simulink model "OWC_rigid"  (R2021b)
settings: Solver=ode45  StartTime=0  StopTime=500  FixedStep=0.01  MaxStep=0.01  RelTol=1e-3  EnableMultiTasking=on
values from neighbouring files (symbols this model uses):
  controlTimestep = 5    [wecSimInputFile.m]
  fExcTimestep = .05    (= 0.05)    [wecSimInputFile.m]
  simu = simulationClass()    [wecSimInputFile.m]
  Z = waveAmplitude * sin(waveFrequency * X) .* cos(waveFrequency * Y)    [userDefinedFunctions.m]
undefined symbols (not defined in the file or in its folder): airChamber, body, constraint, geometry, hydroData, MoorDyn, mooring, pto, turb, WECSim_Lib_Moorings, X, Y
libraries: simulink x6, sm_lib x5, WECSim_Lib_Body_Elements x3, nesl_utility x2, WECSim_Lib_Constraints x1, WECSim_Lib_Frames x1, WECSim_Lib_PTOs x1
settings Model: Creator=mlawson  LastModifiedBy=mshabara
settings SolverCC: ZeroCrossControl=DisableAll  AlgebraicLoopSolver=LineSearch  AutoInsertRateTranBlk=on
settings DataIOCC: SaveFormat=Array  SaveOutput=off  SaveTime=off  ReturnWorkspaceOutputs=off
settings OptimizationCC: LifeSpan=inf  SimCompilerOptimization=on
settings DebuggingCC: MergeDetectMultiDrivingBlocksExec=none  SolverPrmCheckMsg=warning  AllowSymbolicDim=off  StateNameClashWarn=warning  SFUnexpectedBacktrackingDiag=warning  SFNoUnconditionalDefaultTransitionDiag=warning  SFExecutionAtInitializationDiag=none  ArithmeticOperatorsInVariantConditions=warning
settings HardwareCC: ProdBitPerPointer=32  ProdBitPerSizeT=32  ProdBitPerPtrDiffT=32  ProdLargestAtomicFloat=None  ProdIntDivRoundTo=Undefined  ProdEndianess=Unspecified  ProdWordSize=32  ProdHWDeviceType=32-bit Generic
settings ModelReferenceCC: PropagateSignalLabelsOutOfModel=off
settings SFSimCC: SimUseLocalCustomCode=off  CustomCodeUndefinedFunction=UseInterfaceOnly
settings RTWCC: RTWUseLocalCustomCode=off  DLArmComputeVersion=20.02.1
settings CodeAppCC: StateflowObjectComments=on
settings GRTTargetCC: TargetLangStandard=C89/C90 (ANSI)
settings ConfigComp: CovMetricSettings=dw  CovSaveCumulativeToWorkspaceVar=on  CovSaveSingleToWorkspaceVar=on  CovExternalEMLEnable=off  CovSFcnEnable=off
settings SimscapeCC: SimscapeNormalizeSystem=off
settings ConfigurationSet: Description=SimMechanics 2G
settings ExplorerConfigSet: SimMechanicsOpenEditorOnUpdate=off  InternalSimMechanicsExplorerSettings="<ExplorerConfiguration><canonicalview>default</canonicalview><TilePanel><TileInfo><Tiles Columns=\"1\" Count=\"1\" Rows=\"1\"><Column Left=\"2\" Weight=\"1\"/><Column Left=\"1335\"/><Row Top=\"2\" Weight=\"1\"/><Row Top=\"911\"/><Tile Height=\"1\" Width=\"1\" X=\"0\" Y=\"0\"/></Tiles></TileInfo><SceneInfo><SceneViewer><BGColor><R>0.60000002384185791</R><G>0.60000002384185791</G><B>0.60000002384185791</B></BGColor><Camera><Position><X>365.37645888990272</X><Y>-369.82486814446582</Y><Z>359.64809521743916</Z></Position><Center><X>-6.7351450971904585</X><Y>2.2867358426280204</Y><Z>-12.463508769654169</Z></Center><Up><X>-0.40824829046386307</X><Y>0.40824829046386307</Y><Z>0.81649658092772615</Z></Up><Left>-57.820127362122818</Left><Right>57.820127362122818</Right><Bottom>-38.308817187253304</Bottom><Top>38.308817187253304</Top></Camera></SceneViewer></SceneInfo></TilePanel></ExplorerConfiguration>"

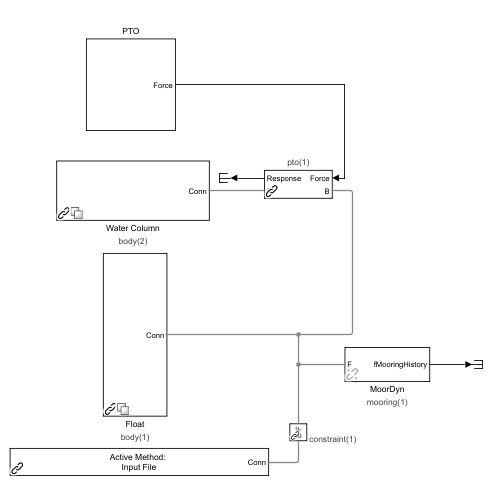
[thumbnail: Simulink's stored preview of the top-level diagram]
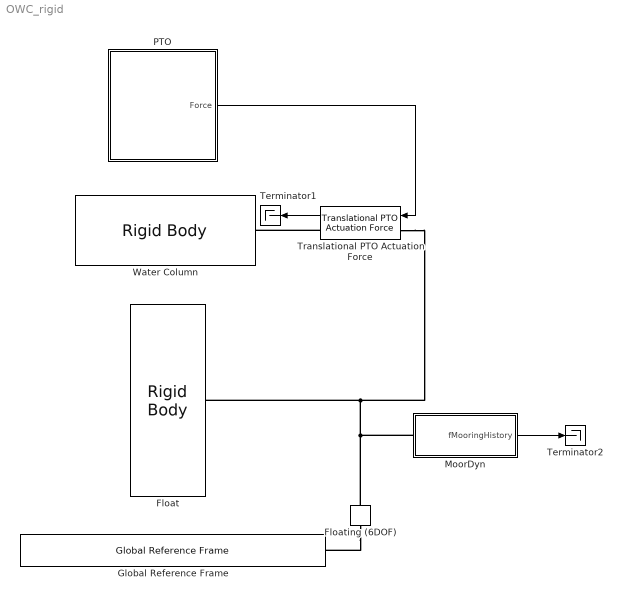
== system OWC_rigid ==
  Float : WECSim_Lib_Body_Elements/Rigid Body  body=body(1)  h5File=hydroData/*.h5  geometryFile=geometry/*.stl  mass=0  inertia=0 0 0  inertiaProducts=0 0 0  nonHydro=0  nonlinearHydro=0  centerGravity=0 0 0  centerBuoyancy=0 0 0  dof=6  volume=0  QTFs=0  displacement=0 0 0  axis=0 1 0  angle=0  option=0  cd=0 0 0  ca=0 0 0  area=0 0 0  VME=0  rgME=0 0 0  z=0 0 1
      settings: SourceProductName=WEC-Sim
  Floating (6DOF) : WECSim_Lib_Constraints/Floating (6DOF)  constraint=constraint(1)  loc="0  0  0"  displacement=0 0 0  y=0 1 0  z=0 0 1  upperLimitSpecify=off  upperLimitBound=0  upperLimitTransitionRegionWidth=0  upperLimitStiffness=0  upperLimitDamping=0  lowerLimitSpecify=off  lowerLimitBound=0  lowerLimitTransitionRegionWidth=0  lowerLimitStiffness=0  lowerLimitDamping=0
      settings: AttributesFormatString=%<constraint>
  Global Reference Frame : WECSim_Lib_Frames/Global Reference Frame  waves=waves  simu=simu  InputMethod=Input File  InputFile=wecSimInputFile.m  mode=normal  explorer=off  solver=ode4  startTime=0  rampTime=100  endTime=400  dt=0.1  cicEndTime=60  stateSpace=0  WaveClass=regular  height=2.5  period=8  elevationFile=NOT DEFINED  spectrumFile=NOT DEFINED  direction=0  spread=1  spectrumType=NOT DEFINED  phaseSeed=0  option=EqualEnergy
      settings: SourceProductName=WEC-Sim
  MoorDyn : Subsystem  AncestorBlock=WECSim_Lib_Moorings/MoorDyn  mask(MoorDyn){mooring=mooring(1), InputFileText=Global Reference Frame option "Use Input File" is selected., MooringRef=0  0  0, moorDynNodes=0, moorDynLines=0}
      mask prompts: mooring "Mooring Name:"; MooringRef "Reference Location [m]:"; moorDynNodes "Number of MoorDyn Nodes:"; moorDynLines "Number of MoorDyn Lines:"
      mask help:
      | A mooring body that applies stiffness, damping and pretensions forces to the follower using a MoorDyn simulation. The response of the mooring body is relative to the global reference frame.
      |
      | The variable name input below must be 'mooring(i)' where i=1,2,...
      | mooring(i) must be defined in the input file with the following fields:
      |
      |     .name (required)
      |             String.
      |             Mooring name. Must comply with Matlab's variable naming rules.
      |     .location (optional)
      |             3x1 vector [x y z] in meters.
      |             Mooring location. Default = [0 0 0]
      |     .initial (optional)
      |             Struct
      |             Contains the initial position, angle and axis of the mooring body.
      |     .initial.displacement (optional)
      |             3x1 vector [x y z] in meters.
      |             Initial linear displacement from the ref position. Default = [0 0 0]
      |             This can can be set directly or with the setInitDisp() method.
      |     .initial.axis (optional)
      |             3x1 vector [x y z]
      |             Initial angular displacement axis. Default = [0 1 0]
      |             This can can be set directly or with the setInitDisp() method.
      |     .initial.angle (optional)
      |             Float.
      |             Initial angular displacement angle about axis in radians. Default = [0 0 0]
      |             This can can be set directly or with the setInitDisp() method.
      |     .moorDynLines (optional)
      |             Float.
      |             Number of lines for MoorDyn to use. Default = 0
      |     .moorDynNodes (optional)
      |             moorDynLines x 1 vector.
      |             Specifies the number of nodes per line in MoorDyn. Default = []
      mask init:
      | if exist('mooring','var')
      |     % toWorkSpace: outputs
      |     h=[gcb '/To Workspace'];
      |     responseName=['mooring' num2str(mooring.number) '_out'];
      |     set_param(h,'VariableName',responseName);
      | end
      | mooring.moorDyn = 1;
      settings: AttributesFormatString=%<mooring>
      mask Help:
      | A mooring body that applies stiffness, damping and pretensions forces to the follower using a MoorDyn simulation. The response of the mooring body is relative to the global reference frame.
      | 
      | The variable name input below must be 'mooring(i)' where i=1,2,...
      | mooring(i) must be defined in the input file with the following fields:
      | 
      |     .name (required)
      |             String.
      |             Mooring name. Must comply with Matlab's variable naming rules.
      |     .location (optional)
      |             3x1 vector [x y z] in meters.
      |             Mooring location. Default = [0 0 0]
      |     .initial (optional)
      |             Struct
      |             Contains the initial position, angle and axis of the mooring body.
      |     .initial.displacement (optional)
      |             3x1 vector [x y z] in meters.
      |             Initial linear displacement from the ref position. Default = [0 0 0]
      |             This can can be set directly or with the setInitDisp() method.
      |     .initial.axis (optional)
      |             3x1 vector [x y z]
      |             Initial angular displacement axis. Default = [0 1 0]
      |             This can can be set directly or with the setInitDisp() method.
      |     .initial.angle (optional)
      |             Float.
      |             Initial angular displacement angle about axis in radians. Default = [0 0 0]
      |             This can can be set directly or with the setInitDisp() method.
      |     .moorDynLines (optional)
      |             Float.
      |             Number of lines for MoorDyn to use. Default = 0
      |     .moorDynNodes (optional)
      |             moorDynLines x 1 vector.
      |             Specifies the number of nodes per line in MoorDyn. Default = []
      mask DialogControl InputFileGroup Prompt: Input File
      mask DialogControl CustomParameterGroup Prompt: Custom Parameters
  PTO : Subsystem
  Terminator1 : Terminator
  Terminator2 : Terminator
  Translational PTO Actuation Force : WECSim_Lib_PTOs/Translational PTO Actuation Force  pto=pto(1)  loc="0  0  0"  stiffness=0  damping=0  equilibriumPosition=0  pretension=0  displacement=0 0 0  y=0 1 0  z=0 0 1  upperLimitSpecify=off  upperLimitBound=0  upperLimitTransitionRegionWidth=0  upperLimitStiffness=0  upperLimitDamping=0  lowerLimitSpecify=off  lowerLimitBound=0  lowerLimitTransitionRegionWidth=0  lowerLimitStiffness=0  lowerLimitDamping=0
      settings: AttributesFormatString=%<pto>
  Water Column : WECSim_Lib_Body_Elements/Rigid Body  body=body(2)  h5File=hydroData/*.h5  geometryFile=geometry/*.stl  mass=0  inertia=0 0 0  inertiaProducts=0 0 0  nonHydro=0  nonlinearHydro=0  centerGravity=0 0 0  centerBuoyancy=0 0 0  dof=6  volume=0  QTFs=0  displacement=0 0 0  axis=0 1 0  angle=0  option=0  cd=0 0 0  ca=0 0 0  area=0 0 0  VME=0  rgME=0 0 0  z=0 0 1
      settings: SourceProductName=WEC-Sim
  wires:
  MoorDyn/1(fMooringHistory) -> Terminator2/1
  Translational PTO Actuation Force/1 -> Terminator1/1
  PTO/1(Force) -> Translational PTO Actuation Force/1
  connections:
  Floating (6DOF)/LConn1 -- Global Reference Frame/RConn1
  MoorDyn/LConn1 -- Floating (6DOF)/RConn1 -- Translational PTO Actuation Force/LConn1 -- Float/RConn1
  Translational PTO Actuation Force/RConn1 -- Water Column/RConn1

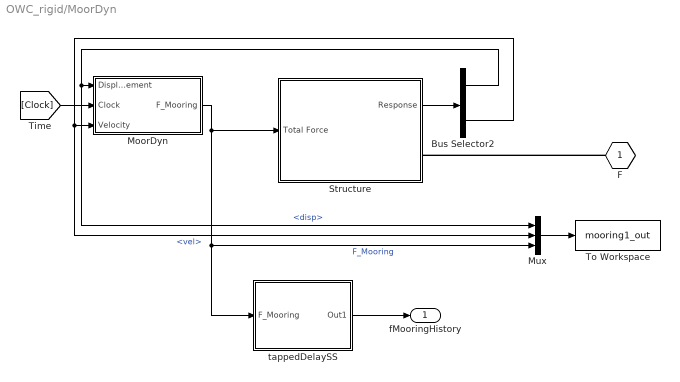
== system OWC_rigid/MoorDyn ==
  Bus Selector2 : BusSelector  OutputSignals=disp,vel
  MoorDyn : Subsystem  VariantControl=sv_moorDyn
  Mux : Mux  Inputs=3
  Structure : Subsystem
  To Workspace : ToWorkspace  VariableName=mooring1_out  SaveFormat=Structure With Time  SampleTime=simu.dtOut
  tappedDelaySS : Subsystem
  F : PMIOPort  Side=Left
  fMooringHistory : Outport
  wires:
  Mux/1 -> To Workspace/1
  Bus Selector2/2 -> MoorDyn/3(Velocity), Mux/2  "<vel>"
  Bus Selector2/1 -> MoorDyn/1(Displacement), Mux/1  "<disp>"
  [Clock] -> MoorDyn/2(Clock)
  MoorDyn/1(F_Mooring) -> Structure/1(Total Force), tappedDelaySS/1(F_Mooring), Mux/3  "F_Mooring"
  Structure/1(Response) -> Bus Selector2/1
  tappedDelaySS/1(Out1) -> fMooringHistory/1
  connections:
  F/RConn1 -- Structure/RConn1

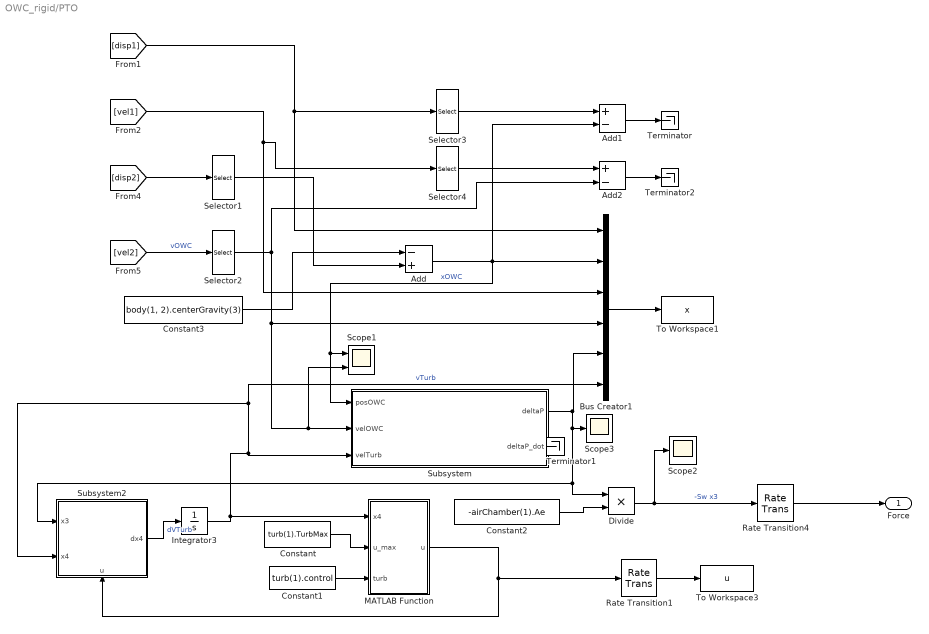
== system OWC_rigid/PTO ==
  Add : Sum  Inputs=-+
  Add1 : Sum  Inputs=+-
  Add2 : Sum  Inputs=+-
  Bus Creator1 : BusCreator  Inputs=6
  Constant : Constant  Value=turb(1).TurbMax
  Constant1 : Constant  Value=turb(1).control
  Constant2 : Constant  Value=-airChamber(1).Ae
  Constant3 : Constant  Value=body(1, 2).centerGravity(3)
  Divide : Product  Inputs=**
  Integrator3 : Integrator  InitialCondition=150
  MATLAB Function : MATLAB Function  TreatAsAtomicUnit=on
  Rate Transition1 : RateTransition  OutPortSampleTimeOpt=Inherit  OutPortSampleTime=controlTimestep
  Rate Transition4 : RateTransition  OutPortSampleTimeOpt=Inherit  OutPortSampleTime=controlTimestep
  Scope1 : Scope  NumInputPorts=2
  Scope2 : Scope
  Scope3 : Scope
  Selector{1..4} (4 alike) : Selector  InputPortWidth=6  IndexOptions=Index vector (dialog)  Indices=3  OutputSizes=1
  Subsystem : Subsystem
  Subsystem2 : Subsystem
      settings: PortSchema="{\"entries\":[{\"content\":{\"sides\":[{\"content\":{\"connectorIds\":[\"In1\",\"In2\"]},\"type\":\"ConnectorPlacement.EquallySpacedRectSide\",\"uuid\":\"efec6f39-391f-477f-a643-1e99d464e6c9\"},{\"content\":{\"connectorIds\":[\"Out1\"],\"side\":\"RIGHT\"},\"type\":\"ConnectorPlacement.EquallySpacedRectSide\",\"uuid\":\"68a722c2-da75-45d7-a9d9-103b5c3e9ffd\"},{\"content\":{\"side\":\"TOP\"},\"type\":\"ConnectorPlacement.EquallySpacedRectSide\",\"uuid\":\"48f59770-5dc2-4659-ad88-cf2781bc51ce\"},{\"content\":{\"connectorIds\":[\"In3\"],\"side\":\"BOTTOM\"},\"type\":\"ConnectorPlacement.EquallySpacedRectSide\",\"uuid\":\"c0a46e7f-e317-4642-bc2a-fe57f83b9e65\"}]},\"type\":\"ConnectorPlacement.EquallySpacedConnector\",\"uuid\":\"2c5b99db-9399-4220-bed2-b879f6d394f4\"}],\"packageUris\":[\"http://schema.mathworks.com/mf0/Connector/R2020b\"],\"version\":\"1.0\"}"
  Terminator : Terminator
  Terminator1 : Terminator
  Terminator2 : Terminator
  To Workspace1 : ToWorkspace  VariableName=x  SaveFormat=Timeseries  SampleTime=-1
  To Workspace3 : ToWorkspace  VariableName=u  SaveFormat=Timeseries  SampleTime=-1
  Force : Outport
  wires:
  Divide/1 -> Scope2/1, Rate Transition4/1  "-Sw x3"
  Add1/1 -> Terminator/1
  [vel1] -> Bus Creator1/3, Selector4/1
  Bus Creator1/1 -> To Workspace1/1
  Constant3/1 -> Add/1
  Add2/1 -> Terminator2/1
  Constant1/1 -> MATLAB Function/3(turb)
  Constant/1 -> MATLAB Function/2(u_max)
  [disp1] -> Bus Creator1/1, Selector3/1
  Subsystem2/1(dx4) -> Integrator3/1  "dVTurb"
  [vel2] -> Selector2/1  "vOWC"
  [disp2] -> Selector1/1
  Integrator3/1 -> Bus Creator1/6, Subsystem2/2(x4), Subsystem/3(velTurb), MATLAB Function/1(x4)  "vTurb"
  Selector3/1 -> Add1/1
  Rate Transition4/1 -> Force/1
  Selector4/1 -> Add2/1
  Add/1 -> Subsystem/1(posOWC), Scope1/1, Add1/2, Bus Creator1/2  "xOWC"
  Subsystem/1(deltaP) -> Scope3/1, Divide/1, Subsystem2/1(x3), Bus Creator1/5
  Subsystem/2(deltaP_dot) -> Terminator1/1
  Constant2/1 -> Divide/2
  Selector1/1 -> Add/2
  Selector2/1 -> Add2/2, Bus Creator1/4, Scope1/2, Subsystem/2(velOWC)
  Rate Transition1/1 -> To Workspace3/1
  MATLAB Function/1(u) -> Rate Transition1/1, Subsystem2/3(u)

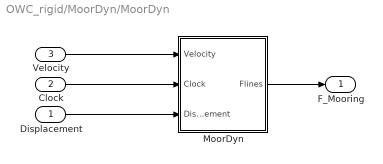
== system OWC_rigid/MoorDyn/MoorDyn ==
  Displacement : Inport
  Clock : Inport  Port=2
  Velocity : Inport  Port=3
  MoorDyn : Subsystem  InitFcn=|  StopFcn=|
      InitFcn=|
      | % Initialize MoorDyn Lib (Windows:dll or OSX:dylib)
      | disp('---------------Starting MoorDyn-----------')
      | 
      | if libisloaded('libmoordyn')
      |     calllib('libmoordyn', 'MoorDynClose');
      |     unloadlibrary libmoordyn;
      | end
      | 
      | if ismac
      |     loadlibrary('libmoordyn.dylib','MoorDyn.h');
      | elseif ispc
      |     loadlibrary('libmoordyn.dll','MoorDyn.h');
      | elseif isunix
      |     loadlibrary('libmoordyn.so','MoorDyn.h');
      | else
      |     disp('Cannot run MoorDyn in this platform');
      | end
      | 
      | calllib('libmoordyn', 'MoorDynInit', mooring.orientation, [0 0 0 0 0 0], mooring.moorDynInputFile);
      | disp('MoorDyn Initialized. Now time stepping...')
      StopFcn=|
      | calllib('libmoordyn', 'MoorDynClose');
      | unloadlibrary libmoordyn;
      settings: CloseFcn=|
      | calllib('libmoordyn', 'MoorDynClose');
      | unloadlibrary libmoordyn;
  F_Mooring : Outport
  wires:
  Velocity/1 -> MoorDyn/1(Velocity)
  Displacement/1 -> MoorDyn/3(Displacement)
  Clock/1 -> MoorDyn/2(Clock)
  MoorDyn/1(Flines) -> F_Mooring/1

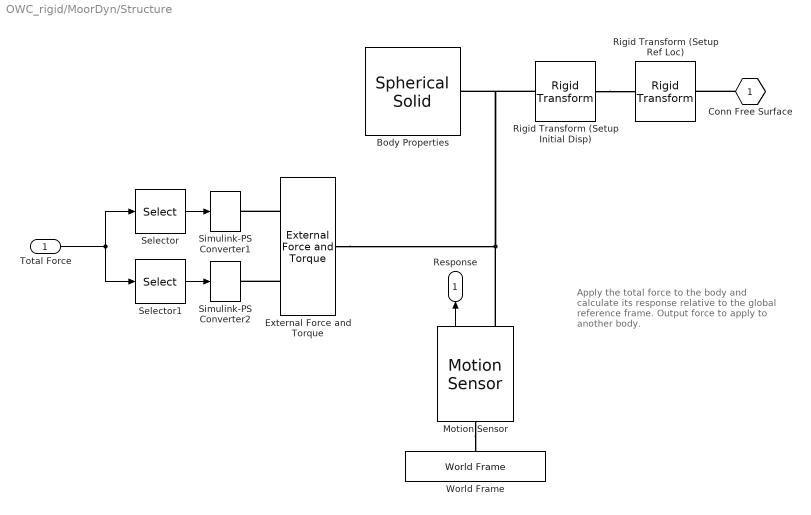
== system OWC_rigid/MoorDyn/Structure ==
  note: Apply the total force to the body and calculate its response relative to the global reference frame.
      |
      | Output force to apply to another body.
  Total Force : Inport
  Body Properties : sm_lib/Body Elements/Spherical Solid  SphereRadius=1  SphereRadiusUnits=m  ExportEntireGeometry=off  InertiaType=Custom  BasedOnType=Density  Density=1000  DensityUnits=kg/(m^3)  Mass=0  MassUnits=kg  CenterOfMass=[0 0 0]  CenterOfMassUnits=m  MomentsOfInertia=[0 0 0]  MomentsOfInertiaUnits=kg*m^2  ProductsOfInertia=[0 0 0]  ProductsOfInertiaUnits=kg*m^2  GraphicType=None  MarkerShape=Sphere  MarkerSize=10  GraphicVisPropType=SimpleVisualProperties  GraphicDiffuseColor=[0 1 0]  GraphicOpacity=1  GraphicSpecularColor=[0.5 0.5 0.5 1.0]  GraphicAmbientColor=[0.15 0.15 0.15 1.0]  GraphicEmissiveColor=[0.0 0.0 0.0 1.0]  GraphicShininess=75  DoExposeReferenceFrame=on  SerializedFrames=<Frames/>
  External Force and Torque : sm_lib/Forces and Torques/External Force and Torque  EnableForceX=off  EnableForceY=off  EnableForceZ=off  EnableForce=on  ForceResolutionFrame=World  EnableTorqueX=off  EnableTorqueY=off  EnableTorqueZ=off  EnableTorque=on  TorqueResolutionFrame=World
  Motion Sensor : WECSim_Lib_Body_Elements/Rigid Body/Hydrodynamic Body/Structure/Motion Sensor  SystemSampleTime=-1  VariantActivationTime=update diagram  Latency=0  AutoFrameSizeCalculation=off
  Rigid Transform (Setup Initial Disp) : sm_lib/Frames and Transforms/Rigid Transform  RotationMethod=ArbitraryAxis  FollAlignAxisA=+X  BaseAlignAxisA=+Y  FollAlignAxisB=+Y  BaseAlignAxisB=+Z  RotationStandardAxis=+Y  RotationAngle=mooring.initial.angle  RotationAngleUnits=rad  RotationArbitraryAxis=mooring.initial.axis  RotationSequenceAxes=FollowerAxes  RotationSequence=XYX  RotationSequenceAngles=[0 0 0]  RotationSequenceAnglesUnits=deg  RotationMatrix=[1 0 0; 0 1 0; 0 0 1]  Quaternion=[1 0 0 0]  TranslationMethod=Cartesian  TranslationCartesianOffset=mooring.initial.displacement  TranslationCartesianOffsetUnits=m  TranslationStandardAxis=+Z  TranslationStandardOffset=0  TranslationStandardOffsetUnits=m  TranslationROffset=0  TranslationROffsetUnits=m  TranslationThetaOffset=0  TranslationThetaOffsetUnits=deg  TranslationZOffset=0  TranslationZOffsetUnits=m
  Rigid Transform (Setup Ref Loc) : sm_lib/Frames and Transforms/Rigid Transform  RotationMethod=None  FollAlignAxisA=+X  BaseAlignAxisA=+Y  FollAlignAxisB=+Y  BaseAlignAxisB=+Z  RotationStandardAxis=+Y  RotationAngle=0.05  RotationAngleUnits=rad  RotationArbitraryAxis=[0.57735026918962584 0.57735026918962584 0.57735026918962584]  RotationSequenceAxes=FollowerAxes  RotationSequence=XYX  RotationSequenceAngles=[0 0 0]  RotationSequenceAnglesUnits=deg  RotationMatrix=[1 0 0; 0 1 0; 0 0 1]  Quaternion=[1 0 0 0]  TranslationMethod=Cartesian  TranslationCartesianOffset=mooring.location  TranslationCartesianOffsetUnits=m  TranslationStandardAxis=+Z  TranslationStandardOffset=0  TranslationStandardOffsetUnits=m  TranslationROffset=0  TranslationROffsetUnits=m  TranslationThetaOffset=0  TranslationThetaOffsetUnits=deg  TranslationZOffset=0  TranslationZOffsetUnits=m
  Selector : Selector  InputPortWidth=6  IndexOptions=Index vector (dialog)  Indices=[1:3]  OutputSizes=1
  Selector1 : Selector  InputPortWidth=6  IndexOptions=Index vector (dialog)  Indices=[4:6]  OutputSizes=1
  Simulink-PS Converter1 : nesl_utility/Simulink-PS Converter  PhysicalDomain=network_engine_domain  SubClassName=ps_input  LeftPortType=input  RightPortType=output  PseudoPeriodic=off  Frequencies=[]  NoiseDistribution=none  NoiseParameters=[]  Unit=1  AffineConversion=off  FilteringAndDerivatives=zero  SimscapeFilterOrder=1  InputFilterTimeConstant=0.001  UdotUserProvided=1
  Simulink-PS Converter2 : nesl_utility/Simulink-PS Converter  PhysicalDomain=network_engine_domain  SubClassName=ps_input  LeftPortType=input  RightPortType=output  PseudoPeriodic=off  Frequencies=[]  NoiseDistribution=none  NoiseParameters=[]  Unit=1  AffineConversion=off  FilteringAndDerivatives=zero  SimscapeFilterOrder=1  InputFilterTimeConstant=0.001  UdotUserProvided=1
  World Frame : sm_lib/Frames and Transforms/World Frame
  Conn Free Surface : PMIOPort  Side=Right
  Response : Outport
  wires:
  Motion Sensor/1 -> Response/1
  Selector1/1 -> Simulink-PS Converter2/1
  Selector/1 -> Simulink-PS Converter1/1
  Total Force/1 -> Selector/1, Selector1/1
  connections:
  Motion Sensor/LConn1 -- World Frame/RConn1
  Rigid Transform (Setup Initial Disp)/LConn1 -- Rigid Transform (Setup Ref Loc)/RConn1
  Conn Free Surface/RConn1 -- Rigid Transform (Setup Ref Loc)/LConn1
  External Force and Torque/RConn1 -- Motion Sensor/RConn1 -- Body Properties/RConn1 -- Rigid Transform (Setup Initial Disp)/RConn1
  External Force and Torque/LConn2 -- Simulink-PS Converter2/RConn1
  External Force and Torque/LConn1 -- Simulink-PS Converter1/RConn1

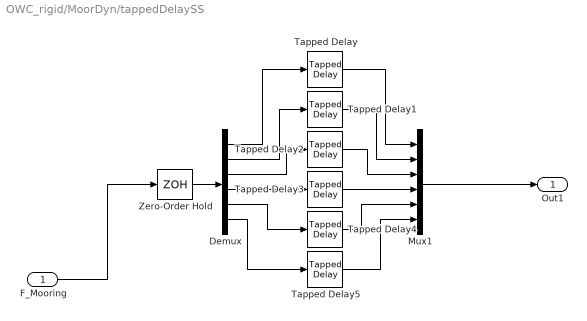
== system OWC_rigid/MoorDyn/tappedDelaySS ==
  F_Mooring : Inport
  Demux : Demux  Outputs=6
  Mux1 : Mux  Inputs=6
  Tapped Delay{,1..5} (6 alike) : simulink/Discrete/Tapped Delay  vinit=0  samptime=-1  NumDelays=controlTimestep/fExcTimestep+1  DelayOrder=Oldest  includeCurrent=off
  Zero-Order Hold : ZeroOrderHold  SampleTime=fExcTimestep
  Out1 : Outport
  wires:
  Demux/6 -> Tapped Delay5/1
  Tapped Delay5/1 -> Mux1/6
  Tapped Delay3/1 -> Mux1/4
  Zero-Order Hold/1 -> Demux/1
  Tapped Delay4/1 -> Mux1/5
  Demux/1 -> Tapped Delay/1
  Tapped Delay2/1 -> Mux1/3
  Tapped Delay1/1 -> Mux1/2
  Tapped Delay/1 -> Mux1/1
  Demux/4 -> Tapped Delay3/1
  Demux/2 -> Tapped Delay1/1
  Demux/3 -> Tapped Delay2/1
  Demux/5 -> Tapped Delay4/1
  Mux1/1 -> Out1/1
  F_Mooring/1 -> Zero-Order Hold/1

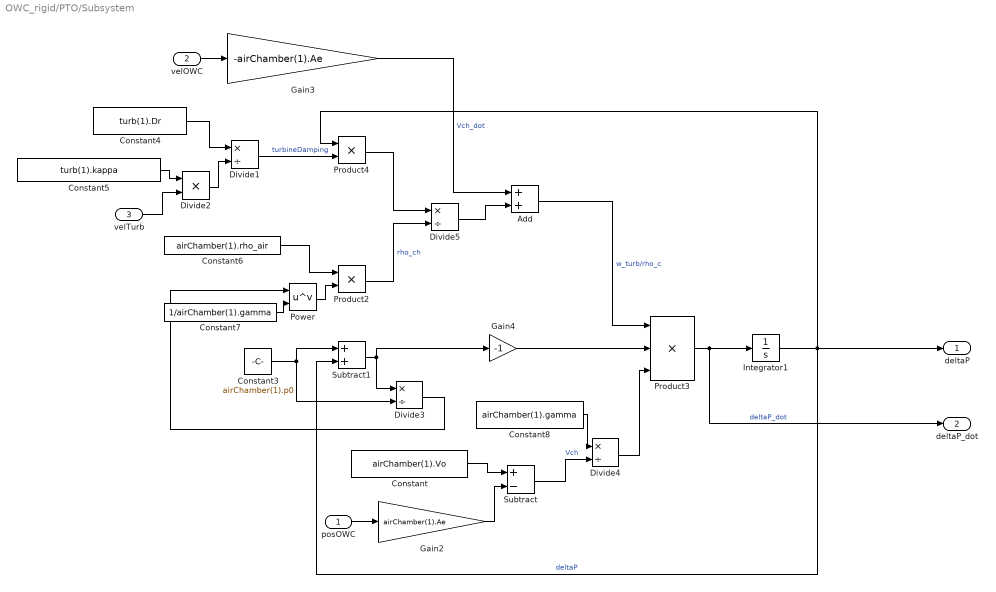
== system OWC_rigid/PTO/Subsystem ==
  posOWC : Inport
  velOWC : Inport  Port=2
  velTurb : Inport  Port=3
  Add : Sum
  Constant : Constant  Value=airChamber(1).Vo
  Constant3 : Constant  Value=airChamber(1).p0
  Constant4 : Constant  Value=turb(1).Dr
  Constant5 : Constant  Value=turb(1).kappa
  Constant6 : Constant  Value=airChamber(1).rho_air
  Constant7 : Constant  Value=1/airChamber(1).gamma
  Constant8 : Constant  Value=airChamber(1).gamma
  Divide{1,3..5} (4 alike) : Product  Inputs=*/
  Divide2 : Product  Inputs=**
  Gain2 : Gain  Gain=airChamber(1).Ae
  Gain3 : Gain  Gain=-airChamber(1).Ae
  Gain4 : Gain  Gain=-1
  Integrator1 : Integrator
  Power : Math  Operator=pow  SaturateOnIntegerOverflow=on
  Product2 : Product
  Product3 : Product  Inputs=3
  Product4 : Product
  Subtract : Sum  Inputs=+-
  Subtract1 : Sum
  deltaP : Outport
  deltaP_dot : Outport  Port=2
  wires:
  Add/1 -> Product3/1  "w_turb/rho_c"
  Constant7/1 -> Power/2
  Constant/1 -> Subtract/1
  Constant3/1 -> Subtract1/1, Divide3/2
  Constant4/1 -> Divide1/1
  Divide3/1 -> Power/1
  Subtract/1 -> Divide4/2  "Vch"
  Gain2/1 -> Subtract/2
  Divide4/1 -> Product3/3
  Product4/1 -> Divide5/1
  velTurb/1 -> Divide2/2
  Divide5/1 -> Add/2
  Integrator1/1 -> Product4/1, deltaP/1, Subtract1/2  "deltaP"
  Subtract1/1 -> Divide3/1, Gain4/1
  velOWC/1 -> Gain3/1
  Constant8/1 -> Divide4/1
  Gain3/1 -> Add/1  "Vch_dot"
  Gain4/1 -> Product3/2
  Product3/1 -> deltaP_dot/1, Integrator1/1  "deltaP_dot"
  Constant6/1 -> Product2/1
  Divide1/1 -> Product4/2  "turbineDamping"
  Divide2/1 -> Divide1/2
  Power/1 -> Product2/2
  Product2/1 -> Divide5/2  "rho_ch"
  Constant5/1 -> Divide2/1
  posOWC/1 -> Gain2/1

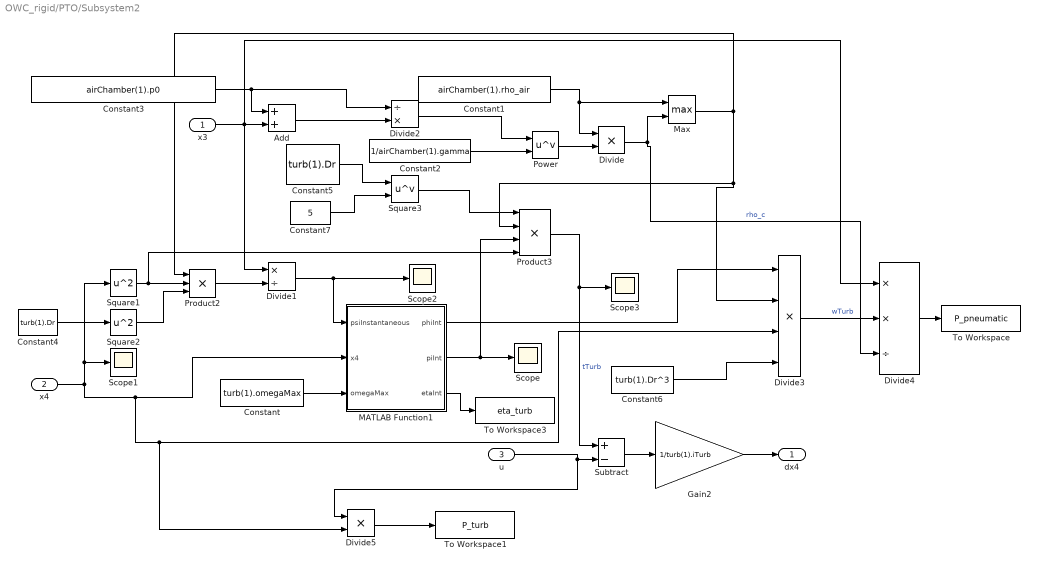
== system OWC_rigid/PTO/Subsystem2 ==
  x3 : Inport
  x4 : Inport  Port=2
  u : Inport  Port=3
  Add : Sum
  Constant : Constant  Value=turb(1).omegaMax
  Constant1 : Constant  Value=airChamber(1).rho_air
  Constant2 : Constant  Value=1/airChamber(1).gamma
  Constant3 : Constant  Value=airChamber(1).p0
  Constant4 : Constant  Value=turb(1).Dr
  Constant5 : Constant  Value=turb(1).Dr
  Constant6 : Constant  Value=turb(1).Dr^3
  Constant7 : Constant  Value=5
  Divide : Product  Inputs=**
  Divide1 : Product  Inputs=*/
  Divide2 : Product  Inputs=/*
  Divide3 : Product  Inputs=****
  Divide4 : Product  Inputs=**/
  Divide5 : Product  Inputs=**
  Gain2 : Gain  Gain=1/turb(1).iTurb
  MATLAB Function1 : MATLAB Function  TreatAsAtomicUnit=on
  Max : MinMax  Function=max  Inputs=2
  Power : Math  Operator=pow  SaturateOnIntegerOverflow=on
  Product2 : Product  Inputs=3
  Product3 : Product  Inputs=4
  Scope{,1..3} (4 alike) : Scope
  Square1 : Math  Operator=square  SaturateOnIntegerOverflow=on
  Square2 : Math  Operator=square  SaturateOnIntegerOverflow=on
  Square3 : Math  Operator=pow  SaturateOnIntegerOverflow=on
  Subtract : Sum  Inputs=+-
  To Workspace : ToWorkspace  VariableName=P_pneumatic  SaveFormat=Timeseries  SampleTime=-1
  To Workspace1 : ToWorkspace  VariableName=P_turb  SaveFormat=Timeseries  SampleTime=-1
  To Workspace3 : ToWorkspace  VariableName=eta_turb  SaveFormat=Timeseries  SampleTime=-1
  dx4 : Outport
  wires:
  Constant4/1 -> Square2/1
  x4/1 -> Square1/1, Scope1/1, Divide5/2, Divide3/3, MATLAB Function1/2(x4)
  Square1/1 -> Product2/2, Product3/4
  Product2/1 -> Divide1/2
  Constant2/1 -> Power/2
  x3/1 -> Divide1/1, Divide4/1, Add/2
  Square2/1 -> Product2/3
  Subtract/1 -> Gain2/1
  Constant3/1 -> Divide2/1, Add/1
  Add/1 -> Divide2/2
  Constant5/1 -> Square3/1
  Constant7/1 -> Square3/2
  Divide1/1 -> MATLAB Function1/1(psiInstantaneous), Scope2/1
  Divide2/1 -> Power/1
  Constant/1 -> MATLAB Function1/3(omegaMax)
  Square3/1 -> Product3/1
  MATLAB Function1/1(phiInt) -> Divide3/1
  MATLAB Function1/2(piInt) -> Scope/1, Product3/3
  Constant1/1 -> Max/1, Divide/1
  Power/1 -> Divide/2
  Product3/1 -> Scope3/1, Subtract/1  "tTurb"
  u/1 -> Divide5/1, Subtract/2
  Divide/1 -> Divide4/3, Max/2  "rho_c"
  Gain2/1 -> dx4/1
  Max/1 -> Product3/2, Divide3/2, Product2/1
  Constant6/1 -> Divide3/4
  Divide3/1 -> Divide4/2  "wTurb"
  Divide4/1 -> To Workspace/1
  Divide5/1 -> To Workspace1/1
  MATLAB Function1/3(etaInt) -> To Workspace3/1

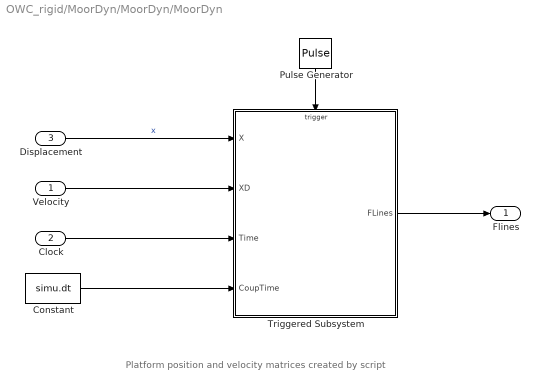
== system OWC_rigid/MoorDyn/MoorDyn/MoorDyn ==
  note: Platform position and velocity matrices created by script
  Velocity : Inport
  Clock : Inport  Port=2
  Displacement : Inport  Port=3
  Constant : Constant  Value=simu.dt
  Pulse Generator : DiscretePulseGenerator  PulseType=Time based  Amplitude=simu.endTime  Period=2*simu.dt  PulseWidth=50
  Triggered Subsystem : Subsystem  TreatAsAtomicUnit=on
  Flines : Outport
  wires:
  Pulse Generator/1 -> Triggered Subsystem/Trigger
  Constant/1 -> Triggered Subsystem/4(CoupTime)
  Velocity/1 -> Triggered Subsystem/2(XD)
  Clock/1 -> Triggered Subsystem/3(Time)
  Triggered Subsystem/1(FLines) -> Flines/1
  Displacement/1 -> Triggered Subsystem/1(X)  "x"

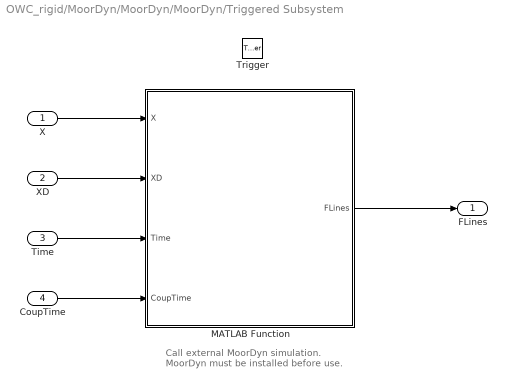
== system OWC_rigid/MoorDyn/MoorDyn/MoorDyn/Triggered Subsystem ==
  note: Call external MoorDyn simulation. MoorDyn must be installed before use.
  X : Inport
  XD : Inport  Port=2
  Time : Inport  Port=3
  CoupTime : Inport  Port=4
  Trigger : TriggerPort  TriggerType=either  VariantControl=(inherit)
  MATLAB Function : MATLAB Function  TreatAsAtomicUnit=on
  FLines : Outport  PortDimensions=6
  wires:
  X/1 -> MATLAB Function/1(X)
  MATLAB Function/1(FLines) -> FLines/1
  XD/1 -> MATLAB Function/2(XD)
  Time/1 -> MATLAB Function/3(Time)
  CoupTime/1 -> MATLAB Function/4(CoupTime)

== matlab function OWC_rigid/PTO/MATLAB Function ==
  data: x4 input; u output; u_max input; turb input
function u = uCalc(x4,u_max, turb)

a = turb(1);
b = turb(2);

u_TEM = a * x4^(b-1);

u = min(u_TEM, u_max);

end

== matlab function OWC_rigid/MoorDyn/MoorDyn/MoorDyn/Triggered Subsystem/MATLAB Function ==
  data: X input; FLines output; XD input; Time input; CoupTime input
function FLines  = MoorDyn_matlab_FCN(X,XD,Time,CoupTime)

FLines = zeros(1,6);
FLines  = MoorDyn_matlab_FCN(X,XD,Time,CoupTime);

end

== matlab function OWC_rigid/PTO/Subsystem2/MATLAB Function1 ==
  data: psiInstantaneous input; phiInt output; piInt output; x4 input; omegaMax input; etaInt output; turb parameter
function [phiInt, piInt, etaInt] = fitCurves(psiInstantaneous, x4, omegaMax, turb)

if x4 > omegaMax
    safeMode = 0;
else
    safeMode = 1;
end

[phiInt, piInt, etaInt] = fitCurves(psiInstantaneous*safeMode, turb(1).psiVec, turb(1).etaTurbVec, turb(1).piVarVec, turb(1).phiVec);

phiInt = phiInt * sign(psiInstantaneous);

end
